simulink model "MBSE_PROJECT1"  (R2019a)
settings: Solver=VariableStepAuto  StartTime=0.0  StopTime=10.0  RelTol=1e-3
undefined symbols (not defined in the file): sigbuilder_block
libraries: simulink x130
(part 3 of 3)

== matlab function MBSE_PROJECT1/MODULES/AirBagSystem/FrontAirBagActivation/WeightSensor ==
  data: driver input; DRIVER output; l_front input; L_FRONT output; l_rear input; r_rear input; L_REAR output; R_REAR output
function [DRIVER,L_FRONT,L_REAR,R_REAR] = fcn(driver, l_front,l_rear,r_rear)
    if (driver==0 && l_front==0 && l_rear==0 && r_rear==1)      %0001
        DRIVER=0;
        L_FRONT=0;
        L_REAR=0;
        R_REAR=1;
    
    elseif (driver==0 && l_front==0 && l_rear==1 && r_rear==0)
        DRIVER=0;
        L_FRONT=0;
        L_REAR=1;
        R_REAR=0;
    
    elseif (driver==0 && l_front==0 && l_rear==1 && r_rear==1)
        DRIVER=0;
        L_FRONT=0;
        L_REAR=1;
        R_REAR=1;

    elseif (driver==0 && l_front==1 && l_rear==0 && r_rear==0)
        DRIVER=0;
        L_FRONT=1;
        L_REAR=0;
        R_REAR=0;
    
    elseif (driver==0 && l_front==1 && l_rear==0 && r_rear==1)
        DRIVER=0;
        L_FRONT=1;
        L_REAR=0;
        R_REAR=1;
    
    elseif (driver==0 && l_front==1 && l_rear==1 && r_rear==0)
        DRIVER=0;
        L_FRONT=1;
        L_REAR=1;
        R_REAR=0;
    
    elseif (driver==0 && l_front==1 && l_rear==1 && r_rear==1)
        DRIVER=0;
        L_FRONT=1;
        L_REAR=1;
        R_REAR=1;
    
    elseif (driver==1 && l_front==0 && l_rear==0 && r_rear==0)
        DRIVER=1;
        L_FRONT=0;
        L_REAR=0;
        R_REAR=0;
    
    elseif (driver==1 && l_front==0 && l_rear==0 && r_rear==1)
        DRIVER=1;
        L_FRONT=0;
        L_REAR=0;
        R_REAR=1;
    
    elseif (driver==1 && l_front==0 && l_rear==1 && r_rear==0)
        DRIVER=1;
        L_FRONT=0;
        L_REAR=1;
        R_REAR=0;
    
    elseif (driver==1 && l_front==0 && l_rear==1 && r_rear==1)
        DRIVER=1;
        L_FRONT=0;
        L_REAR=1;
        R_REAR=1;
    
    elseif (driver==1 && l_front==1 && l_rear==0 && r_rear==0)
        DRIVER=1;
        L_FRONT=1;
        L_REAR=0;
        R_REAR=0;
    
    elseif (driver==1 && l_front==1 && l_rear==0 && r_rear==1)
        DRIVER=1;
        L_FRONT=1;
        L_REAR=0;
        R_REAR=1;
    
    elseif (driver==1 && l_front==1 && l_rear==1 && r_rear==0)
        DRIVER=1;
        L_FRONT=1;
        L_REAR=1;
        R_REAR=0;
    
    elseif (driver==1 && l_front==1 && l_rear==1 && r_rear==1)
        DRIVER=1;
        L_FRONT=1;
        L_REAR=1;
        R_REAR=1;
    
    else
        DRIVER=0;
        L_FRONT=0;
        L_REAR=0;
        R_REAR=0;
    end

== matlab function MBSE_PROJECT1/MODULES/AirBagSystem/SideAirBagActivation/WeightSensor ==
  data: driver input; DRIVER output; l_front input; L_FRONT output; l_rear input; r_rear input; L_REAR output; R_REAR output
function [DRIVER,L_FRONT,L_REAR,R_REAR] = fcn(driver, l_front,l_rear,r_rear)
    if (driver==0 && l_front==0 && l_rear==0 && r_rear==1)      %0001
        DRIVER=0;
        L_FRONT=0;
        L_REAR=0;
        R_REAR=1;
    
    elseif (driver==0 && l_front==0 && l_rear==1 && r_rear==0)
        DRIVER=0;
        L_FRONT=0;
        L_REAR=1;
        R_REAR=0;
    
    elseif (driver==0 && l_front==0 && l_rear==1 && r_rear==1)
        DRIVER=0;
        L_FRONT=0;
        L_REAR=1;
        R_REAR=1;

    elseif (driver==0 && l_front==1 && l_rear==0 && r_rear==0)
        DRIVER=0;
        L_FRONT=1;
        L_REAR=0;
        R_REAR=0;
    
    elseif (driver==0 && l_front==1 && l_rear==0 && r_rear==1)
        DRIVER=0;
        L_FRONT=1;
        L_REAR=0;
        R_REAR=1;
    
    elseif (driver==0 && l_front==1 && l_rear==1 && r_rear==0)
        DRIVER=0;
        L_FRONT=1;
        L_REAR=1;
        R_REAR=0;
    
    elseif (driver==0 && l_front==1 && l_rear==1 && r_rear==1)
        DRIVER=0;
        L_FRONT=1;
        L_REAR=1;
        R_REAR=1;
    
    elseif (driver==1 && l_front==0 && l_rear==0 && r_rear==0)
        DRIVER=1;
        L_FRONT=0;
        L_REAR=0;
        R_REAR=0;
    
    elseif (driver==1 && l_front==0 && l_rear==0 && r_rear==1)
        DRIVER=1;
        L_FRONT=0;
        L_REAR=0;
        R_REAR=1;
    
    elseif (driver==1 && l_front==0 && l_rear==1 && r_rear==0)
        DRIVER=1;
        L_FRONT=0;
        L_REAR=1;
        R_REAR=0;
    
    elseif (driver==1 && l_front==0 && l_rear==1 && r_rear==1)
        DRIVER=1;
        L_FRONT=0;
        L_REAR=1;
        R_REAR=1;
    
    elseif (driver==1 && l_front==1 && l_rear==0 && r_rear==0)
        DRIVER=1;
        L_FRONT=1;
        L_REAR=0;
        R_REAR=0;
    
    elseif (driver==1 && l_front==1 && l_rear==0 && r_rear==1)
        DRIVER=1;
        L_FRONT=1;
        L_REAR=0;
        R_REAR=1;
    
    elseif (driver==1 && l_front==1 && l_rear==1 && r_rear==0)
        DRIVER=1;
        L_FRONT=1;
        L_REAR=1;
        R_REAR=0;
    
    elseif (driver==1 && l_front==1 && l_rear==1 && r_rear==1)
        DRIVER=1;
        L_FRONT=1;
        L_REAR=1;
        R_REAR=1;
    
    else
        DRIVER=0;
        L_FRONT=0;
        L_REAR=0;
        R_REAR=0;
    end

== stateflow chart MBSE_PROJECT1/MODULES/ALARM_SYSTEM/ARMED ==
  state data
  state DELAY_1
    entry:
    data1 = 1;
  state DELAY
    entry:
    count=0;
    count = count + 1;
    data1 = 1;
  data -> DELAY_1 [order 2] : [data==1]
  (default) -> data
  data -> DELAY [order 1] : [data==0]
  DELAY -> DELAY : [count~=30]
  data: data input; data1 output; count local

== stateflow chart MBSE_PROJECT1/MODULES/ALARM_SYSTEM/Main_Alarm/ARMED ==
  state data
  state DELAY_1
    entry:
    data1 = 1;
  state DELAY
    entry:
    count=0;
    count = count + 1;
    data1 = 1;
  data -> DELAY_1 [order 2] : [data==1]
  (default) -> data
  data -> DELAY [order 1] : [data==0]
  DELAY -> DELAY : [count~=30]
  data: data input; data1 output; count local

== stateflow chart MBSE_PROJECT1/MODULES/ALARM_SYSTEM/Main_Alarm/Pre_Alarm ==
  state RKE1
    entry:
  state DELAY_3
    entry:
    data1 = 1;
  state DELAY_2
    entry:
    counter=0;
    counter = counter +1;
    data1 = 0;
  (default) -> RKE1
  RKE1 -> DELAY_3 [order 2] : [data==1]
  RKE1 -> DELAY_2 [order 1] : [data==0]
  DELAY_2 -> DELAY_2 : [counter~=10]
  data: data input; data1 output; counter local

== stateflow chart MBSE_PROJECT1/MODULES/ALARM_SYSTEM/Pre_Alarm ==
  state RKE1
    entry:
  state DELAY_3
    entry:
    data1 = 1;
  state DELAY_2
    entry:
    counter=0;
    counter = counter +1;
    data1 = 0;
  (default) -> RKE1
  RKE1 -> DELAY_3 [order 2] : [data==1]
  RKE1 -> DELAY_2 [order 1] : [data==0]
  DELAY_2 -> DELAY_2 : [counter~=10]
  data: data input; data1 output; counter local
